simulink model "LeftCameraAgent"  (Simulink 6.2)
settings: Solver=ode45  StartTime=0.0  StopTime=10.0  RelTol=1e-3
settings Model: LastModifiedBy=suarezjl
settings DataIOCC: SignalLoggingName=sigsOut
settings HardwareCC: TargetUnknown=on

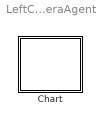
== system LeftCameraAgent ==
  Chart : Stateflow chart

== stateflow chart Chart ==
  state Initial
    \\Sally\HeadTrackingDemo\HeadModule\LeftCameraAgent\FrameGrabber.Initialize()
    \\Sally\HeadTrackingDemo\HeadModule\LeftCameraAgent\FrameGrabber.ObtainImage()
    \\Sally\HeadTrackingDemo\HeadModule\LeftCameraAgent\FrameGrabber.ObtainImage()
    \\Sally\HeadTrackingDemo\HeadModule\LeftCameraAgent\ColorSegmenter.Initialize()
  state Segmentation
    \\Sally\HeadTrackingDemo\HeadModule\LeftCameraAgent\FrameGrabber.ObtainImage()
    \\Sally\HeadTrackingDemo\HeadModule\LeftCameraAgent\ColorSegmenter.DoSegment()
  (default) -> Initial : Start
  Initial -> Segmentation : Always
  Segmentation -> Segmentation : Always
